simulink subsystem "Monitor_Sub"  (R2022b)
settings: Solver=VariableStepAuto  StartTime=0.0  StopTime=10.0  RelTol=1e-3
settings Model: Creator=User  LastModifiedBy=User

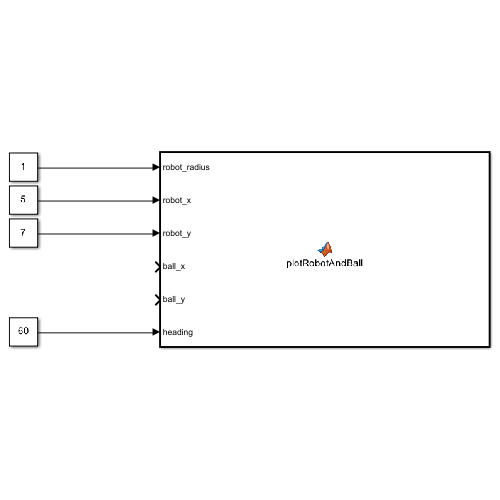
[thumbnail: Simulink's stored preview of the top-level diagram]
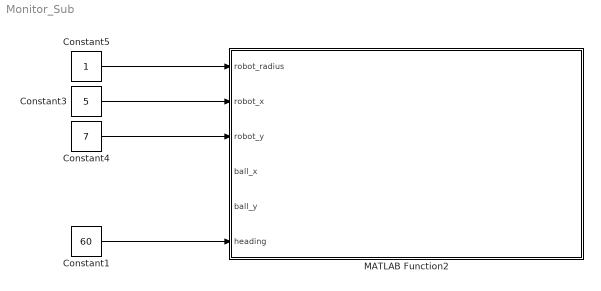
== system Monitor_Sub ==
  Constant1 : Constant  Value=60
  Constant3 : Constant  Value=5
  Constant4 : Constant  Value=7
  Constant5 : Constant
  MATLAB Function2 : MATLAB Function  InitFcn=|  TreatAsAtomicUnit=on
      | figure(1); 
      | clf;
      | hold on; 
      | grid on; 
      | axis([-45,45,-30,30]);
  wires:
  Constant5/1 -> MATLAB Function2/1(robot_radius)
  Constant1/1 -> MATLAB Function2/6(heading)
  Constant4/1 -> MATLAB Function2/3(robot_y)
  Constant3/1 -> MATLAB Function2/2(robot_x)

== matlab function Monitor_Sub/MATLAB Function2 ==
  data: robot_radius input; robot_x input; robot_y input; ball_x input; ball_y input; heading input
function plotRobotAndBall(robot_radius, robot_x, robot_y, ball_x, ball_y, heading)
    figure(1); 
    clf;
    hold on; 
    grid on; 
    axis([-45,45,-30,30]);

    theta = linspace(0, 2*pi, 360);   
    heading_line_length = 4; % L

    % equation of circle for representing robot
    robot_rep_x = robot_radius * cos(theta);
    robot_rep_y = robot_radius * sin(theta);

    heading_line_x = cos((heading*pi)/180) * heading_line_length;
    heading_line_y = sin((heading*pi)/180) * heading_line_length;

    % Draw circle around current location of robot
    plot((robot_rep_x + robot_x), (robot_rep_y + robot_y), 'Color', 'b');
   
    % Draw line from center of robot in the direction of the current heading
    line([robot_x,  robot_x + heading_line_x], [robot_y, robot_y + heading_line_y], 'color', 'b');
    
    % Plot ball
    plot(ball_x, ball_y,'Color','r','Marker','o')

    drawnow();

end
